simulink model "validation_gate"  (Simulink 7.6)
settings: Solver=FixedStepDiscrete  StartTime=0.0  StopTime=0  RelTol=1e-3
values from neighbouring files (symbols this model uses):
  Hedge_Hue = .4    (= 0.4)    [VisionConstants.m]
undefined symbols (not defined in the file or in its folder): Rec, SDTV, strel
libraries: vipconversions x5, simulink x2, vipmorphops x1, vipanalysis x1, viptransforms x1
settings Model: Creator=Thing 1  LastModifiedBy=auvt
settings OptimizationCC: OptimizeModelRefInitCode=on
settings RTWCC: SystemTargetFile=ert.tlc  GenCodeOnly=on  TemplateMakefile=ert_default_tmf  Description=Real-Time Workshop Embedded Coder  GenerateReport=on  ProcessScript=ert_make_rtw_hook  IncludeHyperlinkInReport=on  LaunchReport=on  TargetLang=C++
settings CodeAppCC: IgnoreCustomStorageClasses=off
settings ERTTargetCC: MultiwordLength=2048  GenerateSampleERTMain=on  ERTCustomFileTemplate=example_file_process.tlc  ConvertIfToSwitch=off

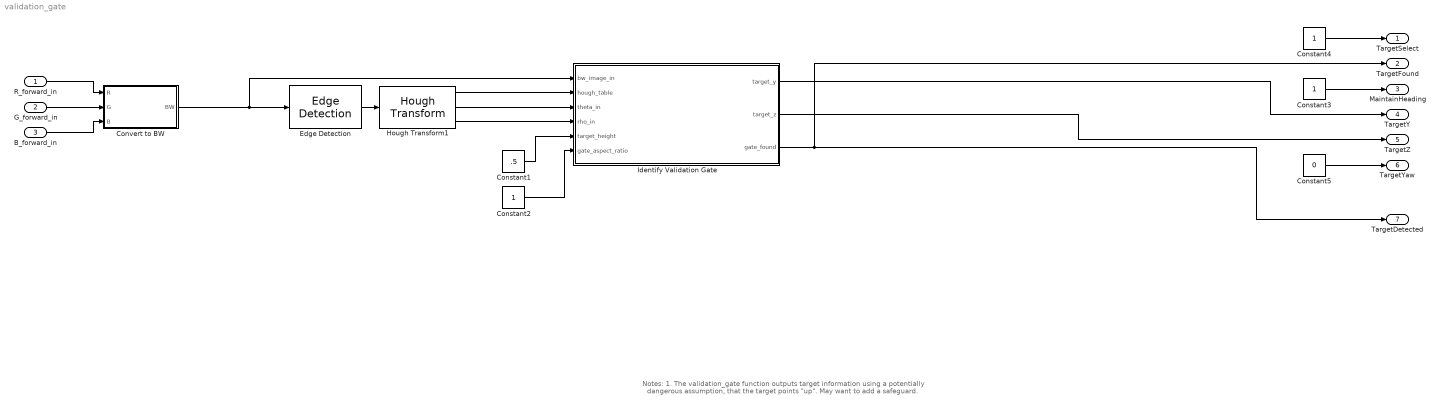
== system validation_gate ==
  note: Notes:
      | 1. The validation_gate function outputs target
      | information using a potentially dangerous
      | assumption, that the target points "up". May
      | want to add a safeguard.
  R_forward_in : Inport  PortDimensions=[160 120]
  G_forward_in : Inport  Port=2  PortDimensions=[160 120]
  B_forward_in : Inport  Port=3  PortDimensions=[160 120]
  Constant1 : Constant  Value=.5  SampleTime=-1
  Constant2 : Constant  SampleTime=-1
  Constant3 : Constant  SampleTime=-1
  Constant4 : Constant  SampleTime=-1
  Constant5 : Constant  Value=0  SampleTime=-1
  Convert to BW : Subsystem
  Edge Detection : vipanalysis/Edge Detection  DialogController=vipDDGCreate  DialogControllerArgs=DataTag3  method=Sobel  outputType=Binary image  userDefinedThreshold=off  thresholdSource=Specify via dialog  threshold=20  thresholdTuning=3  edgeThinning=on  threshold_canny=[0.25 0.60]  autoPercent=70  sigma=1  roundingMode=Floor  overflowMode=off
  Hough Transform1 : viptransforms/Hough Transform  DialogController=vipDDGCreate  DialogControllerArgs=DataTag4  theta_res=pi/180  rho_res=1  out_theta_rho=on  outdtmode=double  firstCoeffMode=Binary point scaling  firstCoeffWordLength=16  firstCoeffFracLength=14  secondCoeffMode=Binary point scaling  secondCoeffWordLength=32  secondCoeffFracLength=16  outputMode=Binary point scaling  outputWordLength=16  outputFracLength=0  accumMode=Binary point scaling  accumWordLength=32  accumFracLength=20  prodOutputMode=Binary point scaling  prodOutputWordLength=32  prodOutputFracLength=20  memoryMode=Binary point scaling  memoryWordLength=32  memoryFracLength=16  roundingMode=Nearest  overflowMode=on
  Identify Validation Gate : Stateflow chart  TreatAsAtomicUnit=on  SystemSampleTime=[1/30 0]
  TargetSelect : Outport  OutDataTypeStr=double
  TargetFound : Outport  Port=2  OutDataTypeStr=double
  MaintainHeading : Outport  Port=3  OutDataTypeStr=double
  TargetY : Outport  Port=4  OutDataTypeStr=double
  TargetZ : Outport  Port=5  OutDataTypeStr=double
  TargetYaw : Outport  Port=6  OutDataTypeStr=double
  TargetDetected : Outport  Port=7  OutDataTypeStr=double
  wires:
  Hough Transform1/1 -> Identify Validation Gate/2(hough_table)
  Hough Transform1/2 -> Identify Validation Gate/3(theta_in)
  Hough Transform1/3 -> Identify Validation Gate/4(rho_in)
  Edge Detection/1 -> Hough Transform1/1
  Constant1/1 -> Identify Validation Gate/5(target_height)
  Constant2/1 -> Identify Validation Gate/6(gate_aspect_ratio)
  R_forward_in/1 -> Convert to BW/1(R)
  G_forward_in/1 -> Convert to BW/2(G)
  B_forward_in/1 -> Convert to BW/3(B)
  Identify Validation Gate/3(gate_found) -> TargetDetected/1, TargetFound/1
  Identify Validation Gate/1(target_y) -> TargetY/1
  Identify Validation Gate/2(target_z) -> TargetZ/1
  Constant3/1 -> MaintainHeading/1
  Constant4/1 -> TargetSelect/1
  Constant5/1 -> TargetYaw/1
  Convert to BW/1(BW) -> Edge Detection/1, Identify Validation Gate/1(bw_image_in)

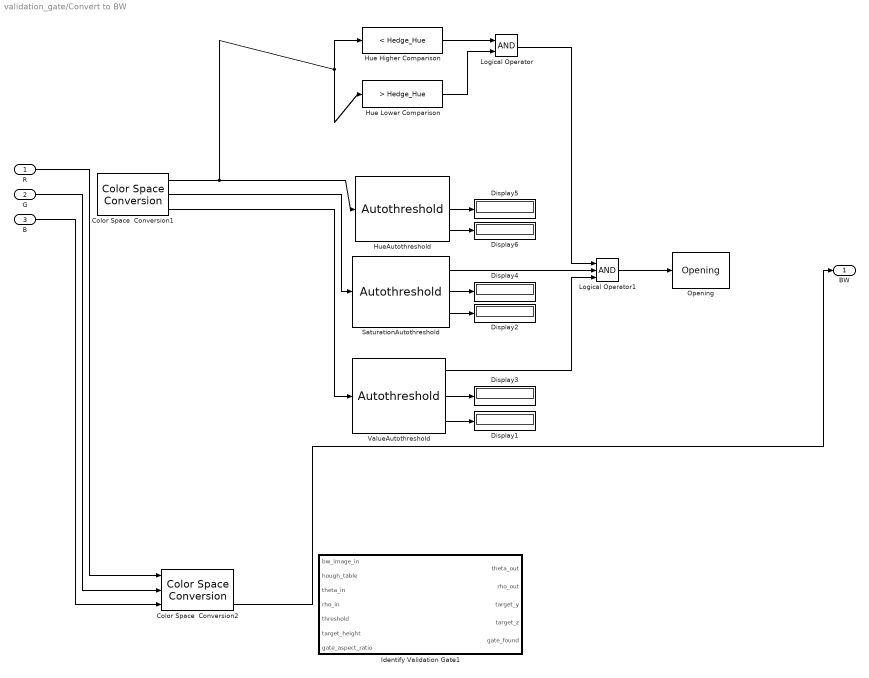
== system validation_gate/Convert to BW ==
  R : Inport  OutDataTypeStr=double
  G : Inport  Port=2  OutDataTypeStr=double
  B : Inport  Port=3  OutDataTypeStr=double
  Color Space  Conversion1 : vipconversions/Color Space  Conversion  conversion=Obsolete  conversionActive=R'G'B' to HSV  wp_str=D65  rec=Rec. 601 (SDTV)  sys=1125/60/2:1  imagePorts=Separate color signals
  Color Space  Conversion2 : vipconversions/Color Space  Conversion  conversion=Obsolete  conversionActive=R'G'B' to HSV  wp_str=D65  rec=Rec. 601 (SDTV)  sys=1125/60/2:1  imagePorts=Separate color signals
  Display{1..6} (6 alike) : Display
  Hue Higher Comparison : simulink/Logic and Bit Operations/Compare To Constant  SystemSampleTime=-1  relop=<  const=Hedge_Hue  LogicOutDataTypeMode=boolean  ZeroCross=off
  Hue Lower Comparison : simulink/Logic and Bit Operations/Compare To Constant  SystemSampleTime=-1  relop=>  const=Hedge_Hue  LogicOutDataTypeMode=boolean  ZeroCross=off
  HueAutothreshold : vipconversions/Autothreshold  DialogController=vipDDGCreate  DialogControllerArgs=DataTag0  operator=>  threshOut=on  effMetricOut=on  userDefinedRange=off  umin=0  umax=255  outOfRngOpt=Warn and saturate  scaleThreshold=off  scaleFactor=1  P1Mode=Specify word length  P1WordLength=32  P1FracLength=30  P2Mode=Specify word length  P2WordLength=32  P2FracLength=22  P3Mode=Specify word length  P3WordLength=32  P3FracLength=14  P4Mode=Binary point scaling  P4WordLength=32  P4FracLength=15  Q1Mode=Specify word length  Q1WordLength=32  Q1FracLength=16  EMMode=Specify word length  EMWordLength=16  EMFracLength=14  roundingMode=Floor  overflowMode=off
  Identify Validation Gate1 : Stateflow chart  TreatAsAtomicUnit=on  SystemSampleTime=[1/30 0]
  Logical Operator : Logic  AllPortsSameDT=off  OutDataTypeStr=fixdt('boolean', 'DataTypeOverride', 'Off')
  Logical Operator1 : Logic  Inputs=3
  Opening : vipmorphops/Opening  nhoodsrc=Specify via dialog  strel=strel('disk',2)
  SaturationAutothreshold : vipconversions/Autothreshold  DialogController=vipDDGCreate  DialogControllerArgs=DataTag1  operator=>  threshOut=on  effMetricOut=on  userDefinedRange=off  umin=0  umax=255  outOfRngOpt=Warn and saturate  scaleThreshold=off  scaleFactor=1  P1Mode=Specify word length  P1WordLength=32  P1FracLength=30  P2Mode=Specify word length  P2WordLength=32  P2FracLength=22  P3Mode=Specify word length  P3WordLength=32  P3FracLength=14  P4Mode=Binary point scaling  P4WordLength=32  P4FracLength=15  Q1Mode=Specify word length  Q1WordLength=32  Q1FracLength=16  EMMode=Specify word length  EMWordLength=16  EMFracLength=14  roundingMode=Floor  overflowMode=off
  ValueAutothreshold : vipconversions/Autothreshold  DialogController=vipDDGCreate  DialogControllerArgs=DataTag2  operator=>  threshOut=on  effMetricOut=on  userDefinedRange=off  umin=0  umax=255  outOfRngOpt=Warn and saturate  scaleThreshold=off  scaleFactor=1  P1Mode=Specify word length  P1WordLength=32  P1FracLength=30  P2Mode=Specify word length  P2WordLength=32  P2FracLength=22  P3Mode=Specify word length  P3WordLength=32  P3FracLength=14  P4Mode=Binary point scaling  P4WordLength=32  P4FracLength=15  Q1Mode=Specify word length  Q1WordLength=32  Q1FracLength=16  EMMode=Specify word length  EMWordLength=16  EMFracLength=14  roundingMode=Floor  overflowMode=off
  BW : Outport
  wires:
  Color Space  Conversion1/2 -> SaturationAutothreshold/1
  Color Space  Conversion1/1 -> HueAutothreshold/1, Hue Lower Comparison/1, Hue Higher Comparison/1
  SaturationAutothreshold/3 -> Display2/1
  Logical Operator/1 -> Logical Operator1/1
  ValueAutothreshold/2 -> Display3/1
  Color Space  Conversion1/3 -> ValueAutothreshold/1
  SaturationAutothreshold/1 -> Logical Operator1/2
  ValueAutothreshold/1 -> Logical Operator1/3
  HueAutothreshold/2 -> Display5/1
  HueAutothreshold/3 -> Display6/1
  SaturationAutothreshold/2 -> Display4/1
  ValueAutothreshold/3 -> Display1/1
  Hue Higher Comparison/1 -> Logical Operator/1
  Hue Lower Comparison/1 -> Logical Operator/2
  Logical Operator1/1 -> Opening/1
  R/1 -> Color Space  Conversion2/1
  G/1 -> Color Space  Conversion2/2
  B/1 -> Color Space  Conversion2/3
  Color Space  Conversion2/3 -> BW/1

== matlab function Identify Validation Gate ==
  data: bw_image_in input double; hough_table input double; target_y output double; target_z output double; gate_found output double; theta_in input double; rho_in input double; target_height input double; gate_aspect_ratio input double
function [target_y, target_z, gate_found] = validation_gate(bw_image_in, hough_table, theta_in, rho_in, target_height, gate_aspect_ratio)
%#eml

% This function attempts to identfiy the validation gate, and returns
%   targeting information, and a true/false gate_found parameter.
%
% 5-29-11
%
% Input
%
%   target_height = fraction of goal post height to aim AUV at
%   gate_aspect_ratio = used to infer unknown points with little extra
%     processing (height/width of large goalpost-shape)
%
% Output
%
% Notes:
%   The hough_table is destroyed in this function (acceptable if
%     hough_table is not an output)
%   Process:
%     1. Identify primary, relatively "long" lines
%     2. 

% Initialize
peak_tol_ratio = .1;  % Fraction of max(rows,cols) of image within which a
%                         peak is assumed to reside; this helps reduce
%                         incorrect line extraction


% Only the (max_num_lines) with the most votes will be considered as
%   candidates for the validation gate
max_num_lines = min( length(rho_in), length(theta_in) );
[rho_length, theta_length] = size(hough_table);
[rows, cols] = size(bw_image_in);



% eps_rho must be at least as big as the gate leg diameter (units of
%   pixels)
eps_rho = .1*max(rows,cols);
% eps_theta is used to distinguish lines as "horizontal" or "vertical";
%   units are radians
eps_theta = 10*pi/180;


% These vectors contain the final three lines that compose the validation gate
rho_gate = zeros(1,3);
theta_gate = zeros(1,3);

% These vectors contain intermediate line information; as lines are
%   eliminated from these vectors, their values are set to zero
rho = zeros(1,max_num_lines);
theta = zeros(1,max_num_lines);





% Identify the most popular max_num_lines lines
i_index = ones(1,max_num_lines);
j_index = ones(1,max_num_lines);

m = 1;
while( m <= max_num_lines )
    
    max_votes = 0;
    for i = 1:rho_length
        for j = 1:theta_length
            if( hough_table(i,j) > max_votes )
                i_index(m) = i;
                j_index(m) = j;
                max_votes = hough_table(i,j);
            end
        end
    end
    
    rho(m) = rho_in(i_index(m));
    theta(m) = theta_in(j_index(m));
    hough_table(i_index(m),j_index(m)) = 0;
    m = m + 1;
    
end


% Eliminate all lines that are not either vertical or horizontal
for i = 1:max_num_lines
    
    condition1 = ( abs(theta(i) - pi/2) <= eps_theta || abs(theta(i) + pi/2) <= eps_theta );  % Vertical line
    condition2 = ( abs(theta(i) - 0) <= eps_theta );  % Horizontal line
    
    if( ~( (condition1 || condition2) && (rho(i) ~= 0) ) )
        rho(i) = 0;
        theta(i) = 0;
    end
    
end




%{
%% The following sorting may not be necessary.
% Sort the rho and theta vectors, keeping track of how many values refer to
%   lines (zero for rho and theta indicate an invalid line)
hold1 = rho;
hold2 = theta;
num_valid_lines = max_num_lines;
for m = 1:max_num_lines
    
    imin = 1;
    lowest_theta = 1000;
    for i = 1:max_num_lines
        if( hold1(i) ~= 0 && hold2(i) < lowest_theta )
            imin = i;
            lowest_theta = hold2(i);
        end
    end
    
    if( lowest_theta ~= 1000 )
        rho(m) = hold1(imin);
        theta(m) = hold2(imin);
        hold1(imin) = 0;
    else
        num_valid_lines = m - 1;
        break;
    end
end
% Set all invalid lines to zeros in rho and theta vectors
for i = (num_valid_lines + 1):max_num_lines
    rho(i) = 0;
    theta(i) = 0;
end
%}



% Effectively generate a small Hough table which contains only values of
%   interest for the validation gate application

rbinv = [0:(2*eps_rho):max(rows, cols)];  % Rho bins for vertical lines
nbinsv = length(rbinv);  % Number of rho bins for vertical lines
ravgv = zeros(1,nbinsv);  % Average rho values for each bin (note that the average value will generally differ slightly than the bin value)
tavgv = zeros(1,nbinsv);  % Average theta values for each bin
vbinv = zeros(1,nbinsv);  % Votes bins for vertical lines

rbinh = [0:(2*eps_rho):max(rows, cols)];
nbinsh = length(rbinh);
ravgh = zeros(1,nbinsh);
tavgh = zeros(1,nbinsh);
vbinh = zeros(1,nbinsh);

for i = 1:max_num_lines
    
    % Consider only lines that are either vertical or horizontal, within
    %   tolerance
    condition1 = ( abs(theta(i) - pi/2) <= eps_theta || abs(theta(i) + pi/2) <= eps_theta );  % Vertical line
    condition2 = ( abs(theta(i) - 0) <= eps_theta );  % Horizontal line
    
    if(condition1)  % Analyze vertical lines
        
        for b = 1:nbinsv

            % Place each rho value into a bin
            if( abs(rho(i) - rbinv(b)) <= eps_rho )
                ravgv(b) = ravgv(b) + rho(i);
                tavgv(b) = tavgv(b) + theta(i);
                vbinv(b) = vbinv(b) + 1;
                break;
            end

        end
        
    elseif(condition2)  % Analyze horizontal lines
        
        theta(i) = theta(i) + pi;
        rho(i) = -rho(i);
        
        for b = 1:nbinsh
            
            % Place each rho value into a bin
            if( abs(rho(i) - rbinh(b)) <= eps_rho )
                ravgh(b) = ravgh(b) + rho(i);
                tavgh(b) = tavgh(b) + theta(i);
                vbinh(b) = vbinh(b) + 1;
                break;
            end
            
        end
        
    end
    
end
    
    
            
%% Extract three lines that fit the criteria for being the validation gate
% Determine the left post as the leftmost vertical line
rmin = 10000;
rmax = -10000;
for b = 1:nbinsv
    if( ravgv(b) < rmin )
        rmin = ravgv(b);
        rho_gate(1) = ravgv(b);
        theta_gate(1) = tavgv(b);
    end
    if( ravgv(b) > rmax )
        rmax = ravgv(b);
        rho_gate(3) = ravgv(b);
        theta_gate(3) = tavgv(b);
    end
end
rmin = 10000;
for b = 1:nbinsh
    if( ravgh(b) < rmin )
        rmin = ravgh(b);
        rho_gate(2) = ravgh(b);
        theta_gate(2) = tavgh(b);
    end
end


%% Compute targeting information
% Compute intersections
r1 = (  ( rho_gate(1)/cos(theta_gate(1)) ) - ( rho_gate(2)/cos(theta_gate(2)) )  )*(  1/( tan(theta_gate(1)) - tan(theta_gate(2)) )  );
c1 = ( 1/cos(theta_gate(1)) )*( rho_gate(1) - r1*sin(theta_gate(1)) );

r3 = (  ( rho_gate(2)/cos(theta_gate(2)) ) - ( rho_gate(3)/cos(theta_gate(3)) )  )*(  1/( tan(theta_gate(2)) - tan(theta_gate(3)) )  );
c3 = ( 1/cos(theta_gate(2)) )*( rho_gate(2) - r3*sin(theta_gate(2)) );

r2 = (r1 + r3)/2;
c2 = (c1 + c3)/2;

% Compute gate width
w = sqrt( (r3 - r1)^2 + (c3 - c1)^2 );

% Form unit vector pointing downward, parallel to gate posts
tavg = ( theta_gate(1) + (theta_gate(2) - pi/2) + theta_gate(3) )/3;
u = [1 1/cos(tavg)];
u = u./norm(u);

% Compute target location
th = target_height*gate_aspect_ratio*w;
r_t = r2 + th*u(1);
c_t = c2 + th*u(2);


% Determine if a gate is present (very simple, potentially inaccurate)
if( sum( (rho_gate == 0) + (theta_gate == 0) ) > 0 )
    
    gate_found = 0;
    target_z = 0;
    target_y = 0;
    
else
    
    gate_found = 1;
    
    % Transform target r, c to global coordinate system
    target_z = r_t - floor(rows/2);
    target_y = c_t - floor(cols/2);
    
end









%{
% Convert rho, theta pairs:
%
%   rho_in can be positive or negative
%   theta_in is a member of [-pi/2, pi/2)
%
%   rho must be positive or zero
%   theta is a member of [0, pi)
for i = 1:max_num_lines
    
    if( theta(i) < 0 )
        theta(i) = theta(i) + pi;
        rho(i) = -rho(i);
    end
%}



%{
% Re-order rho and theta vectors, keeping track of how many values refer to
%   lines (zero for rho and theta indicate an invalid line)
m = 1;
for i = 1:max_num_lines
    if( rho(i) ~= 0 && theta(i) ~= 0 )
        rho(m) = rho(i);
        theta(m) = theta(i);
        m = m + 1;
    end
end

num_valid_lines = m - 1;


% Set all invalid lines to zeros in rho and theta vectors
for i = (num_valid_lines + 1):max_num_lines
    rho(i) = 0;
    theta(i) = 0;
end


% Sort
%}




%{

% Extract the three most popular lines that fit the geometric criteria for
%   the goalpost
rho_gate(1) = rho(1);
theta_gate(1) = theta(1);

m = 2;

%rho_radius = 10;
%theta_radius = 5*pi/180;

for i = 2:max_num_lines
    
    % If rho, theta do not match within tolerance, then store as the next
    %   line
%    if( ( (rho(m) - rho(1))/rho_radius)^2 + ( (theta(m) - theta(1))/theta_radius)^2 > 1 )
    if( abs(rho(i) - rho(i-1)) >= 30 )
        rho_gate(m) = rho(i);
        theta_gate(m) = theta(i);
        m = m + 1;
        if( m > 3 )
            break;
        end
    end
    
end
%}


%{
% Determine whether or not the top three lines constitute the goal post
%   Note that the Simulink block feeding this function keeps theta between
%   +/- pi/2
if( abs(theta_gate(1) - theta_gate(2)) < theta_tol && ( max(theta_gate(1),theta_gate(3)) - min(theta_gate(1),theta_gate(3)) - pi/2 < theta_tol ) )
    gate_found = 1;
    avg_slope = -( 1/tan(theta_gate(1)) + 1/tan(theta_gate(2)) )/2;
    y1 = ( (rho_gate(1)/cos(theta_gate(1))) - (rho_gate(3)/cos(theta_gate(3))) )*( 1/( tan(theta_gate(1)) - tan(theta_gate(3)) ) );
    x1 = ( 1/cos(theta_gate(1)) )*( rho_gate(1) - y1*sin(theta_gate(1)) );
    y2 = ( (rho_gate(2)/cos(theta_gate(2))) - (rho_gate(3)/cos(theta_gate(3))) )*( 1/( tan(theta_gate(2)) - tan(theta_gate(3)) ) );
    x2 = ( 1/cos(theta_gate(2)) )*( rho_gate(2) - y2*sin(theta_gate(2)) );
    
elseif( abs(theta_gate(1) - theta_gate(3)) < theta_tol && ( max(theta_gate(1),theta_gate(2)) - min(theta_gate(1),theta_gate(2)) - pi/2 < theta_tol ) )
    gate_found = 1;
    avg_slope = -( 1/tan(theta_gate(1)) + 1/tan(theta_gate(3)) )/2;
    y1 = ( (rho_gate(1)/cos(theta_gate(1))) - (rho_gate(2)/cos(theta_gate(2))) )*( 1/( tan(theta_gate(1)) - tan(theta_gate(2)) ) );
    x1 = ( 1/cos(theta_gate(1)) )*( rho_gate(1) - y1*sin(theta_gate(1)) );
    y2 = ( (rho_gate(2)/cos(theta_gate(2))) - (rho_gate(3)/cos(theta_gate(3))) )*( 1/( tan(theta_gate(2)) - tan(theta_gate(3)) ) );
    x2 = ( 1/cos(theta_gate(2)) )*( rho_gate(2) - y2*sin(theta_gate(2)) );
    
elseif( abs(theta_gate(2) - theta_gate(3)) < theta_tol && ( max(theta_gate(1),theta_gate(2)) - min(theta_gate(1),theta_gate(2)) - pi/2 < theta_tol ) )
    gate_found = 1;
    avg_slope = -( 1/tan(theta_gate(2)) + 1/tan(theta_gate(3)) )/2;
    y1 = ( (rho_gate(1)/cos(theta_gate(1))) - (rho_gate(2)/cos(theta_gate(2))) )*( 1/( tan(theta_gate(1)) - tan(theta_gate(2)) ) );
    x1 = ( 1/cos(theta_gate(1)) )*( rho_gate(1) - y1*sin(theta_gate(1)) );
    y2 = ( (rho_gate(1)/cos(theta_gate(1))) - (rho_gate(3)/cos(theta_gate(3))) )*( 1/( tan(theta_gate(1)) - tan(theta_gate(3)) ) );
    x2 = ( 1/cos(theta_gate(1)) )*( rho_gate(1) - y2*sin(theta_gate(1)) );
    
else
    gate_found = 0;
    avg_slope = 0;
    
    x1 = 0;
    y1 = 0;
    x2 = 0;
    y2 = 0;
    
end
%}


%{
% Determine targeting information (default to center of viewing area if no
%   gate found)
if( gate_found ~= 0 )
    
    % Determine width and half-height (to center of goal post)
    w = sqrt( (x2 - x1)^2 + (y2 - y1)^2 );
    hh = target_height*gate_aspect_ratio*w;
    
    % Project a line "up" (relative to camera) and determine target
    %   information
    x12 = (x1 + x2)/2;
    y12 = (y1 + y2)/2;
    
    u = [1 -abs(avg_slope)];
    u = u./norm(u);
    
    target_x = x12 + hh*u(1);
    target_y = y12 + hh*u(2);
    
    
    % old code that works, partially
    %phi = atan(avg_slope);
    %target_x = x12 - hh*cos(phi);
    %target_y = y12 - hh*sin(phi);
    
    
    
    
    
    
    %{
    intercept = y12 - avg_slope*x12;
    
    a = avg_slope^2 + 1;
    b = 2*(avg_slope*(intercept - y12) - x12);
    c = x12^2 + (avg_slope - y12)^2 - hh^2;
    
    target_x = real( (-b + sqrt(b^2 - 4*a*c))/(2*a) );
    target_y = avg_slope*target_x + intercept;
    %}
    
    
    
    % Transform target x, y to global coordinate system
    target_z = target_y - floor(rows/2);
    target_y = target_x - floor(cols/2);
    
else
    
    % Default is center of viewing area
    target_x = 0;
    target_y = 0;
    target_z = 0;
    
end
%}





    




return

== matlab function Convert to BW/Identify Validation Gate1 ==
  data: bw_image_in input double; hough_table input double; theta_out output double; rho_out output double; target_y output double; target_z output double; gate_found output double; theta_in input double; rho_in input double; threshold input double; target_height input double; gate_aspect_ratio input double
function [theta_out, rho_out, target_y, target_z, gate_found] = hue_filter(bw_image_in, hough_table, theta_in, rho_in, threshold, target_height, gate_aspect_ratio)
%#eml

% This function attempts to identfiy the validation gate, and returns line
%   information, targeting information, and a true/false gate_found
%   parameter.
%
% 5-29-11
%
% Input
%
%   target_height = fraction of goal post height to aim AUV at
%   gate_aspect_ratio = used to infer unknown points with little extra
%     processing (height/width of large T-shape)
%
% Output
%
% Notes:
%   The hough_table is destroyed in this function (acceptable if
%     hough_table is not an output)
%   Process:
%     1. Identify primary, relatively "long" lines
%     2. 

% Initialize
peak_tol_ratio = .1;  % Fraction of max(rows,cols) of image within which a
%                         peak is assumed to reside; this helps reduce
%                         incorrect line extraction
max_num_lines = 10;  % Considers this many popular lines as candidates

[rho_length, theta_length] = size(hough_table);
[rows, cols] = size(bw_image_in);
rho_tol = .1*max(rows,cols);
theta_tol = 10*pi/180;  % Tolerence within which two slopes are equal (radians)

rho_out = zeros(1,3);
theta_out = zeros(1,3);
rho = zeros(1,max_num_lines);
theta = zeros(1,max_num_lines);



% Apply appropriate threshold
hough_table = hough_table.*( hough_table > threshold );


% Identify the most likely max_num_lines lines
i_index = ones(1,max_num_lines);
j_index = ones(1,max_num_lines);

m = 1;
while( m <= max_num_lines )
    
    max_votes = 0;
    for i = 1:rho_length
        for j = 1:theta_length
            if( hough_table(i,j) > max_votes )
                i_index(m) = i;
                j_index(m) = j;
                max_votes = hough_table(i,j);
            end
        end
    end
    
    rho(m) = rho_in(i_index(m));
    theta(m) = theta_in(j_index(m));
    hough_table(i_index(m),j_index(m)) = 0;
    m = m + 1;
    
end


% Extract the three most popular lines that fit the geometric criteria for
%   the goalpost
rho_out(1) = rho(1);
theta_out(1) = theta(1);

m = 2;

%rho_radius = 10;
%theta_radius = 5*pi/180;

for i = 2:max_num_lines
    
    % If rho, theta do not match within tolerance, then store as the next
    %   line
%    if( ( (rho(m) - rho(1))/rho_radius)^2 + ( (theta(m) - theta(1))/theta_radius)^2 > 1 )
    if( abs(rho(i) - rho(i-1)) >= 30 )
        rho_out(m) = rho(i);
        theta_out(m) = theta(i);
        m = m + 1;
        if( m > 3 )
            break;
        end
    end
    
end


% Determine whether or not the top three lines constitute the goal post
%   Note that the Simulink block feeding this function keeps theta between
%   +/- pi/2
if( abs(theta_out(1) - theta_out(2)) < theta_tol && ( max(theta_out(1),theta_out(3)) - min(theta_out(1),theta_out(3)) - pi/2 < theta_tol ) )
    gate_found = 1;
    avg_slope = -( 1/tan(theta_out(1)) + 1/tan(theta_out(2)) )/2;
    y1 = ( (rho_out(1)/cos(theta_out(1))) - (rho_out(3)/cos(theta_out(3))) )*( 1/( tan(theta_out(1)) - tan(theta_out(3)) ) );
    x1 = ( 1/cos(theta_out(1)) )*( rho_out(1) - y1*sin(theta_out(1)) );
    y2 = ( (rho_out(2)/cos(theta_out(2))) - (rho_out(3)/cos(theta_out(3))) )*( 1/( tan(theta_out(2)) - tan(theta_out(3)) ) );
    x2 = ( 1/cos(theta_out(2)) )*( rho_out(2) - y2*sin(theta_out(2)) );
    
elseif( abs(theta_out(1) - theta_out(3)) < theta_tol && ( max(theta_out(1),theta_out(2)) - min(theta_out(1),theta_out(2)) - pi/2 < theta_tol ) )
    gate_found = 1;
    avg_slope = -( 1/tan(theta_out(1)) + 1/tan(theta_out(3)) )/2;
    y1 = ( (rho_out(1)/cos(theta_out(1))) - (rho_out(2)/cos(theta_out(2))) )*( 1/( tan(theta_out(1)) - tan(theta_out(2)) ) );
    x1 = ( 1/cos(theta_out(1)) )*( rho_out(1) - y1*sin(theta_out(1)) );
    y2 = ( (rho_out(2)/cos(theta_out(2))) - (rho_out(3)/cos(theta_out(3))) )*( 1/( tan(theta_out(2)) - tan(theta_out(3)) ) );
    x2 = ( 1/cos(theta_out(2)) )*( rho_out(2) - y2*sin(theta_out(2)) );
    
elseif( abs(theta_out(2) - theta_out(3)) < theta_tol && ( max(theta_out(1),theta_out(2)) - min(theta_out(1),theta_out(2)) - pi/2 < theta_tol ) )
    gate_found = 1;
    avg_slope = -( 1/tan(theta_out(2)) + 1/tan(theta_out(3)) )/2;
    y1 = ( (rho_out(1)/cos(theta_out(1))) - (rho_out(2)/cos(theta_out(2))) )*( 1/( tan(theta_out(1)) - tan(theta_out(2)) ) );
    x1 = ( 1/cos(theta_out(1)) )*( rho_out(1) - y1*sin(theta_out(1)) );
    y2 = ( (rho_out(1)/cos(theta_out(1))) - (rho_out(3)/cos(theta_out(3))) )*( 1/( tan(theta_out(1)) - tan(theta_out(3)) ) );
    x2 = ( 1/cos(theta_out(1)) )*( rho_out(1) - y2*sin(theta_out(1)) );
    
else
    gate_found = 0;
    avg_slope = 0;
    
    x1 = 0;
    y1 = 0;
    x2 = 0;
    y2 = 0;
    
end


% Determine targeting information (default to center of viewing area if no
%   gate found)
if( gate_found ~= 0 )
    
    % Determine width and half-height (to center of goal post)
    w = sqrt( (x2 - x1)^2 + (y2 - y1)^2 );
    hh = target_height*gate_aspect_ratio*w;
    
    % Project a line "up" (relative to camera) and determine target
    %   information
    x12 = (x1 + x2)/2;
    y12 = (y1 + y2)/2;
    
    u = [1 -abs(avg_slope)];
    u = u./norm(u);
    
    target_x = x12 + hh*u(1);
    target_y = y12 + hh*u(2);
    
    
    % old code that works, partially
    %phi = atan(avg_slope);
    %target_x = x12 - hh*cos(phi);
    %target_y = y12 - hh*sin(phi);
    
    
    
    
    
    
    %{
    intercept = y12 - avg_slope*x12;
    
    a = avg_slope^2 + 1;
    b = 2*(avg_slope*(intercept - y12) - x12);
    c = x12^2 + (avg_slope - y12)^2 - hh^2;
    
    target_x = real( (-b + sqrt(b^2 - 4*a*c))/(2*a) );
    target_y = avg_slope*target_x + intercept;
    %}
    
    
    
    % Transform target x, y to global coordinate system
    target_z = target_y - floor(rows/2);
    target_y = target_x - floor(cols/2);
    
else
    
    % Default is center of viewing area
    target_x = 0;
    target_y = 0;
    target_z = 0;
    
end


return
